simulink model "control_simulink"  (R2015a)
settings: Solver=ode3  StartTime=0.0  StopTime=10  FixedStep=0.001  RelTol=1e-3
values from neighbouring files (symbols this model uses):
  b = -3.15*10^-4    (= -0.000315)    [controlmodeltestspoleplacment.m]    (also in controlwithintegratorsLQR.m; controlwithoutencoderonlyMPUgains.m)
  g = 9.81    [controlmodeltestspoleplacment.m]    (also in controlwithintegratorsLQR.m; controlwithoutencoderonlyMPUgains.m)
  Jb = 0.02    [controlmodeltestspoleplacment.m]    (also in controlwithintegratorsLQR.m = 0.01; controlwithoutencoderonlyMPUgains.m = 0.0015)
  Jw = 8.99*10^-4    (= 0.000899)    [controlmodeltestspoleplacment.m]    (also in controlwithintegratorsLQR.m; controlwithoutencoderonlyMPUgains.m)
  K = place(A,B,[p1, p2, p3,p4])    [controlmodeltestspoleplacment.m]    (also in controlwithintegratorsLQR.m = lqr(A,B,Q,RR); controlwithoutencoderonlyMPUgains.m = lqr(A,B,Q,RR))
  Ke = 0.006    [controlmodeltestspoleplacment.m]    (also in controlwithintegratorsLQR.m; controlwithoutencoderonlyMPUgains.m)
  Km = 0.0018    [controlmodeltestspoleplacment.m]    (also in controlwithintegratorsLQR.m; controlwithoutencoderonlyMPUgains.m)
  L = 0.080    (= 0.08)    [controlmodeltestspoleplacment.m]    (also in controlwithintegratorsLQR.m = 0.11; controlwithoutencoderonlyMPUgains.m = 0.068)
  Mb = 0.562-0.033*2+0.3    (= 0.796)    [controlmodeltestspoleplacment.m]    (also in controlwithintegratorsLQR.m = 0.896; controlwithoutencoderonlyMPUgains.m = 0.396)
  Mw = 0.033    [controlmodeltestspoleplacment.m]    (also in controlwithintegratorsLQR.m; controlwithoutencoderonlyMPUgains.m)
  Nbar = K(1)    [controlmodeltestspoleplacment.m]    (also in controlwithintegratorsLQR.m; controlwithoutencoderonlyMPUgains.m = K(3))
  R = 5.6/48    (= 0.116666666667)    [controlmodeltestspoleplacment.m]    (also in controlwithintegratorsLQR.m; controlwithoutencoderonlyMPUgains.m)
  r = 0.0335    [controlmodeltestspoleplacment.m]    (also in controlwithintegratorsLQR.m; controlwithoutencoderonlyMPUgains.m)
  x_0 = [0 0 0 0]    [controlmodeltestspoleplacment.m]    (also in controlwithintegratorsLQR.m = [0 0 0.1 0 0]; controlwithoutencoderonlyMPUgains.m = [0 0 0.01 0 0])
settings Model: Creator=omaRhagrass  LastModifiedBy=omaRhagrass
settings SolverCC: ZeroCrossControl=DisableAll  ZeroCrossAlgorithm=Adaptive  AlgebraicLoopSolver=LineSearch  PositivePriorityOrder=on  AutoInsertRateTranBlk=on
settings DataIOCC: LimitDataPoints=off

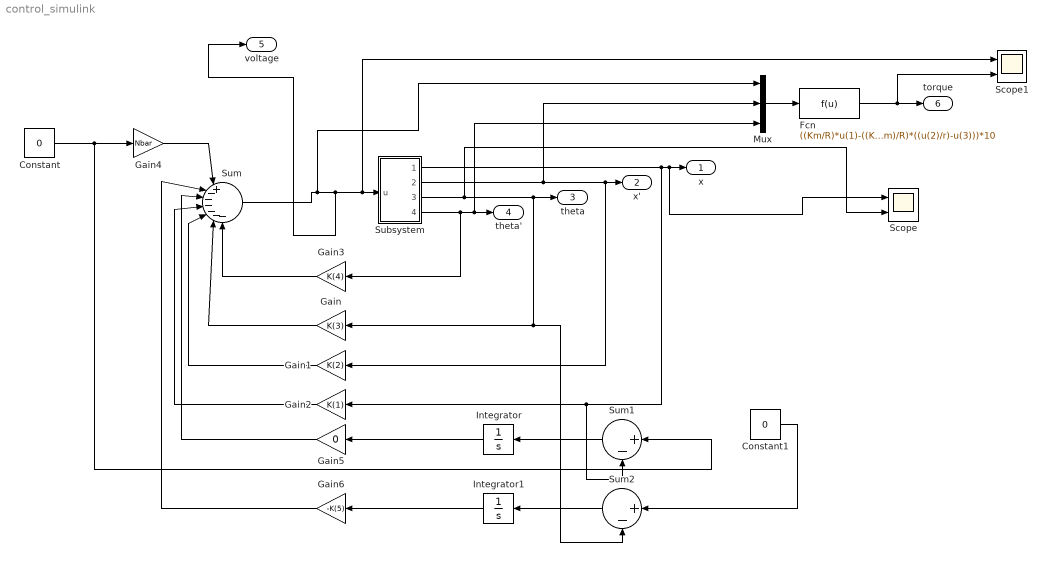
== system control_simulink ==
  Constant : Constant  Value=0
  Constant1 : Constant  Value=0
  Fcn : Fcn  Expr=((Km/R)*u(1)-((Ke*Km)/R)*((u(2)/r)-u(3)))*10
  Gain : Gain  Gain=K(3)
  Gain1 : Gain  Gain=K(2)
  Gain2 : Gain  Gain=K(1)
  Gain3 : Gain  Gain=K(4)
  Gain4 : Gain  Gain=Nbar
  Gain5 : Gain  Gain=0
  Gain6 : Gain  Gain=-K(5)
  Integrator : Integrator
  Integrator1 : Integrator
  Mux : Mux  Inputs=3
  Scope : Scope  NumInputPorts=2
      settings: YMin=-5~-5  YMax=5~5
  Scope1 : Scope  NumInputPorts=2
      settings: YMin=-5~-5  YMax=5~5
  Subsystem : Subsystem
  Sum : Sum  Inputs=|+------
  Sum1 : Sum  Inputs=|+-
  Sum2 : Sum  Inputs=|+-
  "x " : Outport
  "x' " : Outport  Port=2
  "theta " : Outport  Port=3
  "theta' " : Outport  Port=4
  voltage : Outport  Port=5
  "torque " : Outport  Port=6
  wires:
  Subsystem/2(Out2) -> Mux/2, Gain1/1, "x' "/1
  Subsystem/3(Out3) -> Scope/2, Gain/1, Sum2/2, "theta "/1
  Subsystem/4(Out4) -> Gain3/1, Mux/3, "theta' "/1
  Subsystem/1(Out1) -> Sum1/2, Gain2/1, Scope/1, "x "/1
  Constant/1 -> Sum1/1, Gain4/1
  Gain4/1 -> Sum/1
  Gain3/1 -> Sum/7
  Gain/1 -> Sum/6
  Gain1/1 -> Sum/5
  Gain2/1 -> Sum/4
  Gain5/1 -> Sum/3
  Gain6/1 -> Sum/2
  Integrator1/1 -> Gain6/1
  Integrator/1 -> Gain5/1
  Sum1/1 -> Integrator/1
  Sum2/1 -> Integrator1/1
  Sum/1 -> Mux/1, voltage/1, Scope1/1, Subsystem/1("u ")
  Constant1/1 -> Sum2/1
  Mux/1 -> Fcn/1
  Fcn/1 -> Scope1/2, "torque "/1

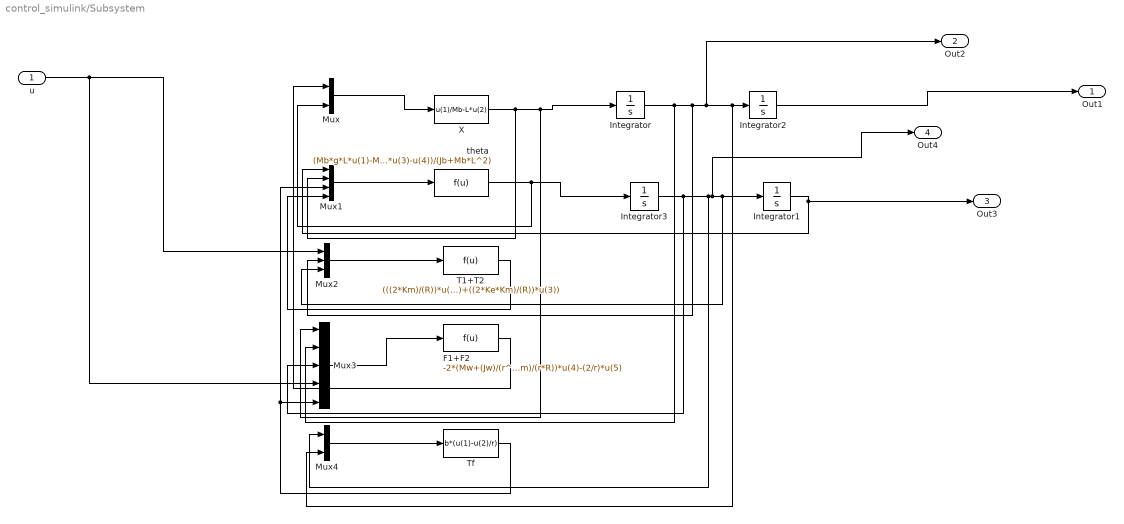
== system control_simulink/Subsystem ==
  "u " : Inport
  "F1+F2 " : Fcn  Expr=-2*(Mw+(Jw)/(r^2))*u(1)-((2*Km*Ke)/(R*(r^2)))*u(2)+((2*Km*Ke)/(R*r))*u(3)+((2*Km)/(r*R))*u(4)-(2/r)*u(5)
  Integrator : Integrator
  Integrator1 : Integrator  InitialCondition=x_0(3)
  Integrator2 : Integrator  InitialCondition=x_0(1)
  Integrator3 : Integrator
  Mux : Mux  Inputs=2
  Mux1 : Mux
  Mux2 : Mux  Inputs=3
  Mux3 : Mux  Inputs=5
  Mux4 : Mux  Inputs=2
  "T1+T2 " : Fcn  Expr=(((2*Km)/(R))*u(1)-((2*Km*Ke)/(R*r))*u(2)+((2*Ke*Km)/(R))*u(3))
  "Tf " : Fcn  Expr=b*(u(1)-u(2)/r)
  X : Fcn  Expr=u(1)/Mb-L*u(2)
  "theta " : Fcn  Expr=(Mb*g*L*u(1)-Mb*L*u(2)+2*u(3)-u(4))/(Jb+Mb*L^2)
  Out1 : Outport
  Out2 : Outport  Port=2
  Out3 : Outport  Port=3
  Out4 : Outport  Port=4
  wires:
  Integrator/1 -> Mux3/2, Mux2/2, Out2/1, Mux4/2, Integrator2/1
  Integrator3/1 -> Mux3/3, Mux4/1, Out4/1, Mux2/3, Integrator1/1
  Mux3/1 -> "F1+F2 "/1
  Mux2/1 -> "T1+T2 "/1
  Mux1/1 -> "theta "/1
  Mux/1 -> X/1
  X/1 -> Mux1/2, Mux3/1, Integrator/1
  "theta "/1 -> Mux/2, Integrator3/1
  "F1+F2 "/1 -> Mux/1
  Mux4/1 -> "Tf "/1
  Integrator1/1 -> Out3/1, Mux1/1
  "Tf "/1 -> Mux3/5, Mux1/3
  "T1+T2 "/1 -> Mux1/4
  "u "/1 -> Mux3/4, Mux2/1
  Integrator2/1 -> Out1/1
